simulink model "TRIGA_model"  (R2017b)
settings: Solver=ode15s  StartTime=0  StopTime=10000  RelTol=1e-2  EnableMultiTasking=on
values from neighbouring files (symbols this model uses):
  A_Frict = (H_Core*F_D)./(2*DEq*(AFlow^2)*Rho_In)    [ReactorModel.m]
  AFlow = 0.06352    [ReactorModel.m]
  Alpha_C = 4*10^-5    (= 4e-05)    [ReactorModel.m]
  Alpha_F = -8.5*10^-5    (= -8.5e-05)    [ReactorModel.m]
  Alpha_V = -2.5e-06    [ReactorModel.m]
  Beta = BetaTOT*Fraction    [ReactorModel.m]
  BetaTOT = 730*10^-5    (= 0.0073)    [ReactorModel.m]
  CCool = CCool*1000    [ReactorModel.m]
  DEq = 4*AFlow/PWet    (= 0.0237633472062)    [ReactorModel.m]
  ESigmaF = U_0*SigmaFiss    (= 0.056935026)    [ReactorModel.m]
  f = 1    [ReactorModel.m]
  GCore_0 = (H_Core*9.81*Rho_In*NuExp.*P0./(A_Frict.*CCool)).^(1/3)    [ReactorModel.m]
  H_Active = 0.381    [ReactorModel.m]
  H_Core = 0.7224    [ReactorModel.m]
  I_0 = (Y_I*SigmaFiss*U_0*Phi_0)/LambdaI    (= 1.16996991958e+14)    [ReactorModel.m]
  KCool = XSteam('tc_pT',Pressure,TCool_0)    [ReactorModel.m]
  Lambda = [3.01 1.14 0.301 0.111 0.0305 0.0124]    [ReactorModel.m]
  LambdaI = 2.87*10^-5    (= 2.87e-05)    [ReactorModel.m]
  LambdaPm = 3.63*10^-6    (= 3.63e-06)    [ReactorModel.m]
  LambdaXe = 2.09*10^-5    (= 2.09e-05)    [ReactorModel.m]
  Life = 60*10^-6    (= 6e-05)    [ReactorModel.m]
  M1 = 7    [ReactorModel.m]
  M3 = 7.6    [ReactorModel.m]
  M_Res = 800    [ReactorModel.m]
  MCool = 22.57    [ReactorModel.m]
  MPool = 18963    [ReactorModel.m]
  Mu = XSteam('my_pT', Pressure, TCool_0)    [ReactorModel.m]
  N_Fuel = 83    [ReactorModel.m]
  N_Mean = 2.43    [ReactorModel.m]
  NuExp = 245*10^-6    (= 0.000245)    [ReactorModel.m]
  P0 = 50000    [ReactorModel.m]
  Phi_0 = P0/(EFiss*ESigmaF*N_Fuel*V_Fuel*10^6)    (= 922945828545)    [ReactorModel.m]
  Pm_0 = (Y_Pm*SigmaFiss*U_0*Phi_0)/LambdaPm    (= 1.55038151024e+14)    [ReactorModel.m]
  Pr = (Mu.*CCool)./KCool    [ReactorModel.m]
  PWet = 2*pi*RCladO*91    (= 10.6920964372)    [ReactorModel.m]
  R_Rod = 0.00089    [ReactorModel.m]
  RCladO = 0.0187    [ReactorModel.m]
  Rho_0 = XSteam('rho_pT', Pressure, TCool_0)    [ReactorModel.m]
  RT_Clad = (log(RCladO/R_CladI))/(2*pi*K_Clad)    [ReactorModel.m]
  RT_Fuel = 1/(8*pi*K_Fuel)    (= 0.00226329555023)    [ReactorModel.m]
  RT_Gap = 1/(2*pi*R_GapO*H_Gap)    (= 0.00348193602083)    [ReactorModel.m]
  SigmaSm = 4.1*10^-20    (= 4.1e-20)    [ReactorModel.m]
  SigmaXe = 2.65*10^-18    (= 2.65e-18)    [ReactorModel.m]
  Sm_0 = (LambdaPm*Pm_0)/(SigmaSm*Phi_0)    (= 1.48725397185e+16)    [ReactorModel.m]
  Step = 1    [ReactorModel.m]
  T_Aq = 15    [ReactorModel.m]
  TCool_0 = TPool_0+(P0./(20*GCore_0.*CCool))    [ReactorModel.m]
  TFuel_0 = (f*P0./K)+TCool_0    [ReactorModel.m]
  TPool_0 = TPool_R+(P0./(MPool*CCool))    [ReactorModel.m]
  TPool_R = 20    [ReactorModel.m]
  W = 0.5    [ReactorModel.m]
  Xe_0 = (Y_Xe*SigmaFiss*U_0*Phi_0 + LambdaI*I_0)/(SigmaXe*Phi_0 + LambdaXe)    (= 1.49163932561e+14)    [ReactorModel.m]
  Y_I = 0.0639    [ReactorModel.m]
  Y_Pm = 0.01071    [ReactorModel.m]
  Y_Xe = 0.00237    [ReactorModel.m]
libraries: simulink x2
settings Model: Creator=dironco  LastModifiedBy=Introini Carolina
settings DataIOCC: LimitDataPoints=on  InspectSignalLogs=on
settings OptimizationCC: LifeSpan=inf
settings DebuggingCC: AllowSymbolicDim=off  SFUnexpectedBacktrackingDiag=warning  SFNoUnconditionalDefaultTransitionDiag=warning  SFExecutionAtInitializationDiag=none
settings ModelReferenceCC: PropagateSignalLabelsOutOfModel=off
settings CodeAppCC: StateflowObjectComments=on
settings GRTTargetCC: TargetLangStandard=C89/C90 (ANSI)
settings ConfigComp: CovMetricSettings=dw  CovHtmlReporting=on  CovSaveCumulativeToWorkspaceVar=on  CovSaveSingleToWorkspaceVar=on  CovExternalEMLEnable=off

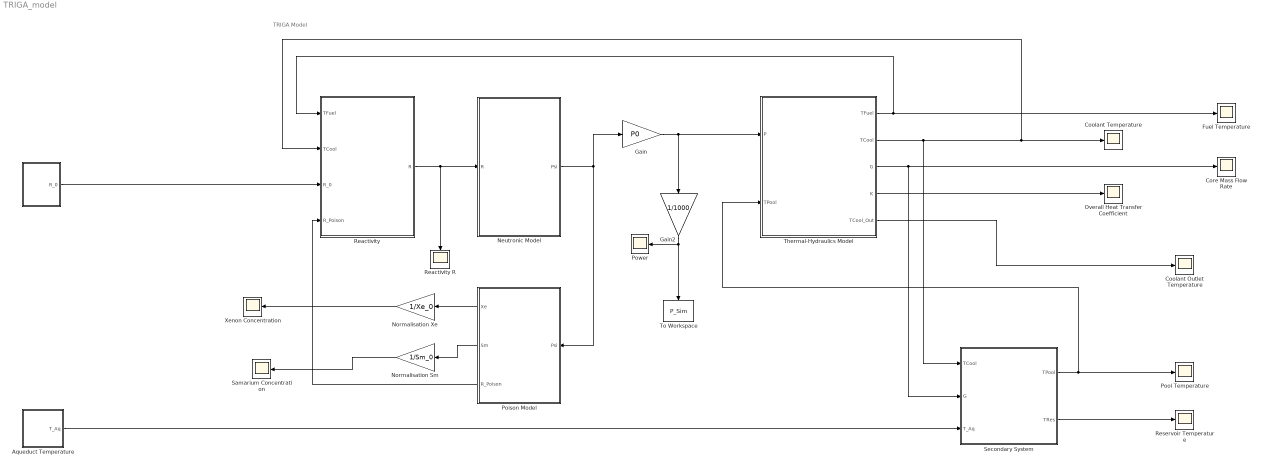
== system TRIGA_model ==
  note: TRIGA Model
  " " : Subsystem  Tag=Input Reactivity
  Aqueduct Temperature : Subsystem
  Coolant Outlet Temperature : Scope
  Coolant Temperature : Scope
  Core Mass Flow Rate : Scope
  Fuel Temperature : Scope
  Gain : Gain  Gain=P0
  Gain2 : Gain  Gain=1/1000
  Neutronic Model : Subsystem
  Normalisation Sm : Gain  Gain=1/Sm_0
  Normalisation Xe : Gain  Gain=1/Xe_0
  Overall Heat Transfer Coefficient : Scope
  Poison Model : Subsystem
  Pool Temperature : Scope
  Power : Scope
  Reactivity : Subsystem
  Reactivity R : Scope
  Reservoir Temperature : Scope
  Samarium Concentration : Scope
  Secondary System : Subsystem
  "Thermal-Hydraulics Model " : Subsystem
  To Workspace : ToWorkspace  VariableName=P_Sim  SaveFormat=Structure With Time  SampleTime=0.1
  Xenon Concentration : Scope
  wires:
  "Thermal-Hydraulics Model "/2(TCool) -> Secondary System/1(TCool), Reactivity/2(TCool), Coolant Temperature/1
  "Thermal-Hydraulics Model "/4(K) -> Overall Heat Transfer Coefficient/1
  Secondary System/1(TPool) -> "Thermal-Hydraulics Model "/2(TPool), Pool Temperature/1
  "Thermal-Hydraulics Model "/1(TFuel) -> Reactivity/1(TFuel), Fuel Temperature/1
  "Thermal-Hydraulics Model "/5(TCool_Out) -> Coolant Outlet Temperature/1
  "Thermal-Hydraulics Model "/3(G) -> Secondary System/2(G), Core Mass Flow Rate/1
  Gain2/1 -> To Workspace/1, Power/1
  Reactivity/1(R) -> Neutronic Model/1(R), Reactivity R/1
  Normalisation Xe/1 -> Xenon Concentration/1
  Normalisation Sm/1 -> Samarium Concentration/1
  Secondary System/2(TRes) -> Reservoir Temperature/1
  Poison Model/1(Xe) -> Normalisation Xe/1
  Poison Model/3(R_Poison) -> Reactivity/4(R_Poison)
  Aqueduct Temperature/1(T_Aq) -> Secondary System/3(T_Aq)
  " "/1(R_0) -> Reactivity/3(R_0)
  Poison Model/2(Sm) -> Normalisation Sm/1
  Gain/1 -> "Thermal-Hydraulics Model "/1(P), Gain2/1
  Neutronic Model/1("Psi ") -> Poison Model/1(Psi), Gain/1

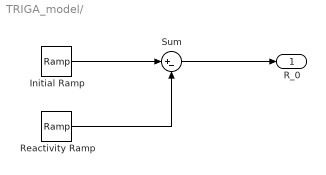
== system TRIGA_model/  ==
  Initial Ramp : simulink/Sources/Ramp  slope=R_Rod/Step  start=50  X0=0
  Reactivity Ramp : simulink/Sources/Ramp  slope=R_Rod/Step  start=Step+50  X0=0
  Sum : Sum  Inputs=|+-
  R_0 : Outport
  wires:
  Reactivity Ramp/1 -> Sum/2
  Initial Ramp/1 -> Sum/1
  Sum/1 -> R_0/1

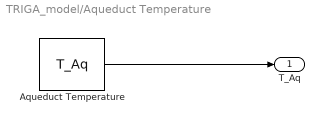
== system TRIGA_model/Aqueduct Temperature ==
  Aqueduct Temperature : Constant  Value=T_Aq
  T_Aq : Outport
  wires:
  Aqueduct Temperature/1 -> T_Aq/1

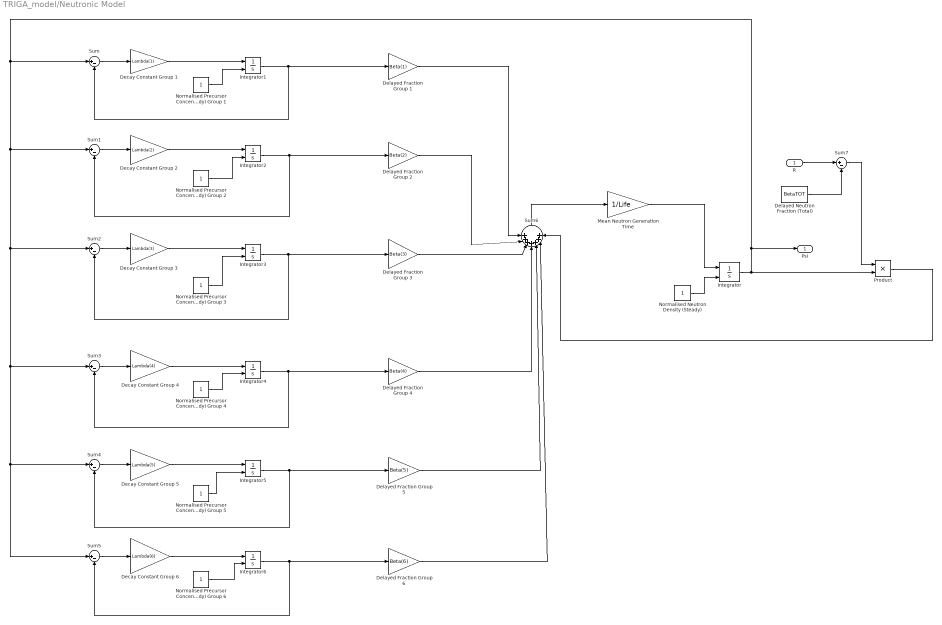
== system TRIGA_model/Neutronic Model ==
  R : Inport
  Decay Constant Group 1 : Gain  Gain=Lambda(1)
  Decay Constant Group 2 : Gain  Gain=Lambda(2)
  Decay Constant Group 3 : Gain  Gain=Lambda(3)
  Decay Constant Group 4 : Gain  Gain=Lambda(4)
  Decay Constant Group 5 : Gain  Gain=Lambda(5)
  Decay Constant Group 6 : Gain  Gain=Lambda(6)
  Delayed Fraction Group 1 : Gain  Gain=Beta(1)
  Delayed Fraction Group 2 : Gain  Gain=Beta(2)
  Delayed Fraction Group 3 : Gain  Gain=Beta(3)
  Delayed Fraction Group 4 : Gain  Gain=Beta(4)
  Delayed Fraction Group 5 : Gain  Gain=Beta(5)
  Delayed Fraction Group 6 : Gain  Gain=Beta(6)
  Delayed Neutron Fraction (Total) : Constant  Value=BetaTOT
  Integrator{,1..6} (7 alike) : Integrator  InitialConditionSource=external
  Mean Neutron Generation Time : Gain  Gain=1/Life
  Normalised Precursor Concentration (Steady) Group {1..6} (6 alike) : Constant
  Normalised Neutron Density (Steady) : Constant
  Product : Product
  Sum{,1..5,7} (7 alike) : Sum  Inputs=|+-
  Sum6 : Sum  Inputs=+++++++
  "Psi " : Outport
  wires:
  Sum1/1 -> Decay Constant Group 2/1
  Sum/1 -> Decay Constant Group 1/1
  Sum3/1 -> Decay Constant Group 4/1
  Sum5/1 -> Decay Constant Group 6/1
  Sum6/1 -> Mean Neutron Generation Time/1
  Integrator1/1 -> Sum/2, Delayed Fraction Group 1/1
  Integrator2/1 -> Sum1/2, Delayed Fraction Group 2/1
  Integrator3/1 -> Sum2/2, Delayed Fraction Group 3/1
  Sum4/1 -> Decay Constant Group 5/1
  Integrator4/1 -> Sum3/2, Delayed Fraction Group 4/1
  Sum2/1 -> Decay Constant Group 3/1
  Integrator5/1 -> Sum4/2, Delayed Fraction Group 5/1
  Delayed Fraction Group 5/1 -> Sum6/5
  Delayed Fraction Group 1/1 -> Sum6/1
  Mean Neutron Generation Time/1 -> Integrator/1
  Delayed Fraction Group 2/1 -> Sum6/2
  Delayed Fraction Group 4/1 -> Sum6/4
  Normalised Precursor Concentration (Steady) Group 5/1 -> Integrator5/2
  Integrator/1 -> Sum3/1, Sum5/1, Sum4/1, Sum2/1, Sum1/1, Sum/1, "Psi "/1, Product/2
  Normalised Precursor Concentration (Steady) Group 3/1 -> Integrator3/2
  Normalised Precursor Concentration (Steady) Group 2/1 -> Integrator2/2
  Normalised Precursor Concentration (Steady) Group 1/1 -> Integrator1/2
  Integrator6/1 -> Delayed Fraction Group 6/1, Sum5/2
  Delayed Fraction Group 6/1 -> Sum6/6
  Normalised Precursor Concentration (Steady) Group 6/1 -> Integrator6/2
  Normalised Precursor Concentration (Steady) Group 4/1 -> Integrator4/2
  Normalised Neutron Density (Steady)/1 -> Integrator/2
  Product/1 -> Sum6/7
  Delayed Fraction Group 3/1 -> Sum6/3
  R/1 -> Sum7/1
  Decay Constant Group 1/1 -> Integrator1/1
  Decay Constant Group 2/1 -> Integrator2/1
  Decay Constant Group 3/1 -> Integrator3/1
  Decay Constant Group 4/1 -> Integrator4/1
  Decay Constant Group 5/1 -> Integrator5/1
  Decay Constant Group 6/1 -> Integrator6/1
  Delayed Neutron Fraction (Total)/1 -> Sum7/2
  Sum7/1 -> Product/1

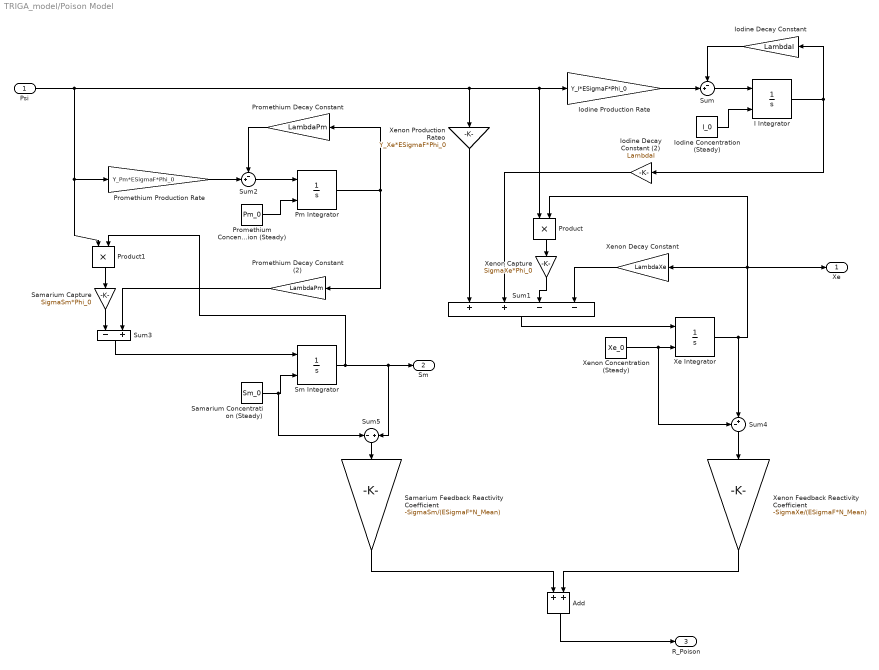
== system TRIGA_model/Poison Model ==
  Psi : Inport
  Add : Sum
  I Integrator : Integrator  InitialConditionSource=external
  Iodine Concentration (Steady) : Constant  Value=I_0
  Iodine Decay Constant : Gain  Gain=LambdaI
  Iodine Decay Constant (2) : Gain  Gain=LambdaI
  Iodine Production Rate : Gain  Gain=Y_I*ESigmaF*Phi_0
  Pm Integrator : Integrator  InitialConditionSource=external
  Product : Product
  Product1 : Product
  Promethium Concentration (Steady) : Constant  Value=Pm_0
  Promethium Decay Constant : Gain  Gain=LambdaPm
  Promethium Decay Constant (2) : Gain  Gain=LambdaPm
  "Promethium Production Rate " : Gain  Gain=Y_Pm*ESigmaF*Phi_0
  Samarium Capture : Gain  Gain=SigmaSm*Phi_0
  Samarium Concentration (Steady) : Constant  Value=Sm_0
  Samarium Feedback Reactivity Coefficient : Gain  Gain=-SigmaSm/(ESigmaF*N_Mean)
  Sm Integrator : Integrator  InitialConditionSource=external
  Sum : Sum  Inputs=-+|
  Sum1 : Sum  Inputs=++--
  Sum2 : Sum  Inputs=-+|
  Sum3 : Sum  Inputs=-+
  Sum4 : Sum  Inputs=-+|
  Sum5 : Sum  Inputs=-+
  Xe Integrator : Integrator  InitialConditionSource=external
  Xenon Capture : Gain  Gain=SigmaXe*Phi_0
  Xenon Feedback Reactivity Coefficient : Gain  Gain=-SigmaXe/(ESigmaF*N_Mean)
  Xenon Production Rateo : Gain  Gain=Y_Xe*ESigmaF*Phi_0
  Xenon Concentration (Steady) : Constant  Value=Xe_0
  Xenon Decay Constant : Gain  Gain=LambdaXe
  Xe : Outport
  Sm : Outport  Port=2
  R_Poison : Outport  Port=3
  wires:
  I Integrator/1 -> Iodine Decay Constant/1, Iodine Decay Constant (2)/1
  Iodine Decay Constant/1 -> Sum/1
  Iodine Concentration (Steady)/1 -> I Integrator/2
  Sum/1 -> I Integrator/1
  Iodine Production Rate/1 -> Sum/2
  Xe Integrator/1 -> Xe/1, Product/2, Xenon Decay Constant/1, Sum4/2
  Xenon Decay Constant/1 -> Sum1/4
  Sum1/1 -> Xe Integrator/1
  Iodine Decay Constant (2)/1 -> Sum1/2
  Xenon Production Rateo/1 -> Sum1/1
  Product/1 -> Xenon Capture/1
  Xenon Capture/1 -> Sum1/3
  Promethium Concentration (Steady)/1 -> Pm Integrator/2
  Psi/1 -> Iodine Production Rate/1, Product/1, Xenon Production Rateo/1, "Promethium Production Rate "/1, Product1/1
  Sum2/1 -> Pm Integrator/1
  Pm Integrator/1 -> Promethium Decay Constant (2)/1, Promethium Decay Constant/1
  Promethium Decay Constant/1 -> Sum2/1
  "Promethium Production Rate "/1 -> Sum2/2
  Sum3/1 -> Sm Integrator/1
  Promethium Decay Constant (2)/1 -> Sum3/2
  Product1/1 -> Samarium Capture/1
  Samarium Capture/1 -> Sum3/1
  Sm Integrator/1 -> Sum5/2, Sm/1, Product1/2
  Samarium Concentration (Steady)/1 -> Sum5/1, Sm Integrator/2
  Sum4/1 -> Xenon Feedback Reactivity Coefficient/1
  Xenon Concentration (Steady)/1 -> Sum4/1, Xe Integrator/2
  Sum5/1 -> Samarium Feedback Reactivity Coefficient/1
  Xenon Feedback Reactivity Coefficient/1 -> Add/2
  Samarium Feedback Reactivity Coefficient/1 -> Add/1
  Add/1 -> R_Poison/1

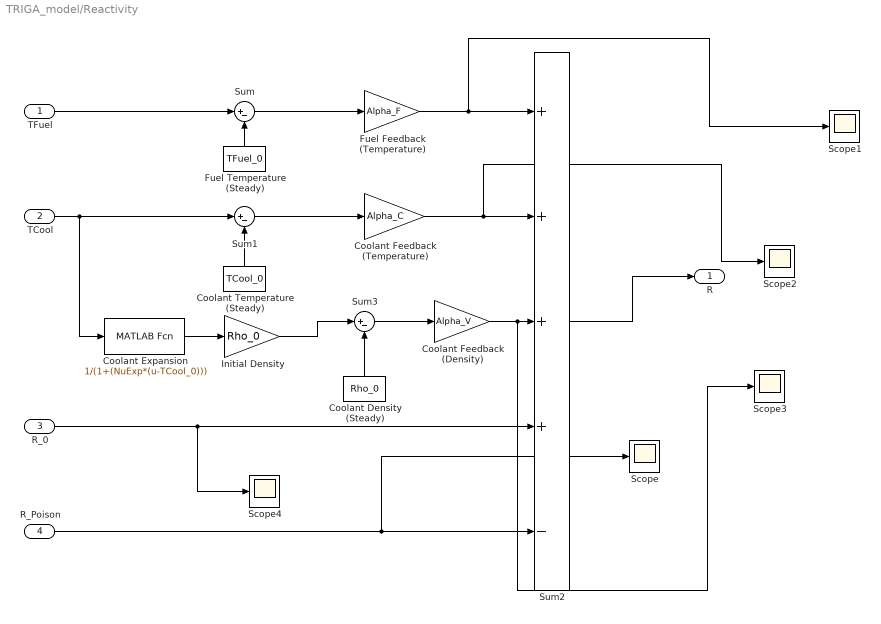
== system TRIGA_model/Reactivity ==
  TFuel : Inport
  TCool : Inport  Port=2
  R_0 : Inport  Port=3
  R_Poison : Inport  Port=4
  Coolant Density (Steady) : Constant  Value=Rho_0
  Coolant Expansion : MATLABFcn  MATLABFcn=1/(1+(NuExp*(u-TCool_0)))
  Coolant Feedback (Density) : Gain  Gain=Alpha_V
  Coolant Feedback (Temperature) : Gain  Gain=Alpha_C
  Coolant Temperature (Steady) : Constant  Value=TCool_0
  Fuel Feedback (Temperature) : Gain  Gain=Alpha_F
  Fuel Temperature (Steady) : Constant  Value=TFuel_0
  Initial Density : Gain  Gain=Rho_0
  Scope{,1..4} (5 alike) : Scope
  Sum : Sum  Inputs=|+-
  Sum1 : Sum  Inputs=|+-
  Sum2 : Sum  Inputs=++++-
  Sum3 : Sum  Inputs=|+-
  R : Outport
  wires:
  Coolant Temperature (Steady)/1 -> Sum1/2
  Sum2/1 -> R/1
  Sum1/1 -> Coolant Feedback (Temperature)/1
  TFuel/1 -> Sum/1
  Sum/1 -> Fuel Feedback (Temperature)/1
  R_0/1 -> Scope4/1, Sum2/4
  Coolant Feedback (Temperature)/1 -> Scope2/1, Sum2/2
  TCool/1 -> Coolant Expansion/1, Sum1/1
  Fuel Temperature (Steady)/1 -> Sum/2
  Fuel Feedback (Temperature)/1 -> Scope1/1, Sum2/1
  R_Poison/1 -> Scope/1, Sum2/5
  Coolant Feedback (Density)/1 -> Scope3/1, Sum2/3
  Coolant Expansion/1 -> Initial Density/1
  Initial Density/1 -> Sum3/1
  Sum3/1 -> Coolant Feedback (Density)/1
  Coolant Density (Steady)/1 -> Sum3/2

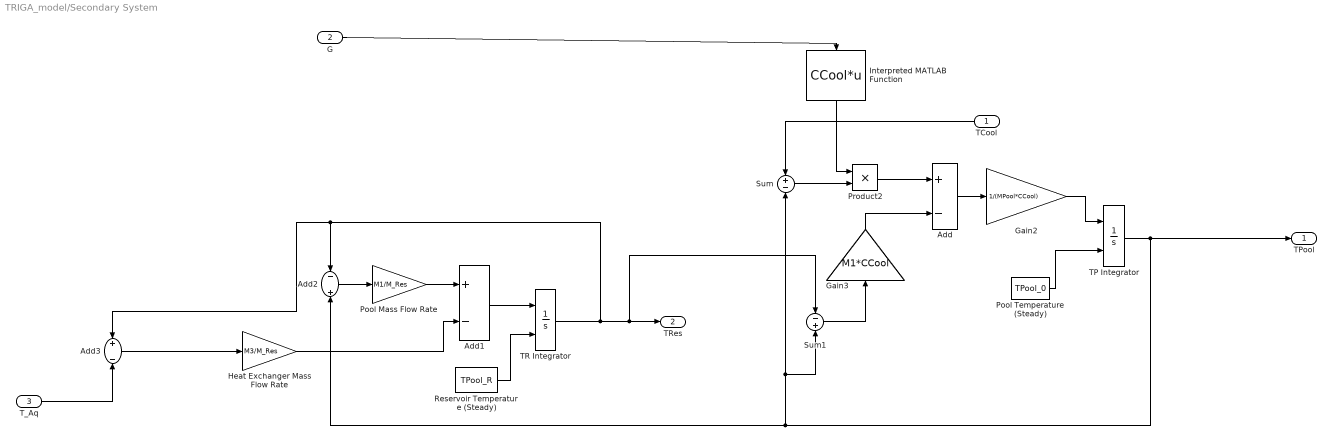
== system TRIGA_model/Secondary System ==
  TCool : Inport
  G : Inport  Port=2
  T_Aq : Inport  Port=3
  Add : Sum  Inputs=+-
  Add1 : Sum  Inputs=+-
  Add2 : Sum  Inputs=-+
  Add3 : Sum  Inputs=+-
  Gain2 : Gain  Gain=1/(MPool*CCool)
  Gain3 : Gain  Gain=M1*CCool
  "Heat Exchanger Mass Flow Rate " : Gain  Gain=M3/M_Res
  Interpreted MATLAB Function : MATLABFcn  MATLABFcn=CCool*u
  Pool Mass Flow Rate : Gain  Gain=M1/M_Res
  Pool Temperature (Steady) : Constant  Value=TPool_0
  Product2 : Product
  Reservoir Temperature (Steady) : Constant  Value=TPool_R
  Sum : Sum  Inputs=+-
  Sum1 : Sum  Inputs=-+
  TP Integrator : Integrator  InitialConditionSource=external
  TR Integrator : Integrator  InitialConditionSource=external
  TPool : Outport
  TRes : Outport  Port=2
  wires:
  Add1/1 -> TR Integrator/1
  Reservoir Temperature (Steady)/1 -> TR Integrator/2
  "Heat Exchanger Mass Flow Rate "/1 -> Add1/2
  Pool Temperature (Steady)/1 -> TP Integrator/2
  Gain2/1 -> TP Integrator/1
  Add3/1 -> "Heat Exchanger Mass Flow Rate "/1
  Interpreted MATLAB Function/1 -> Product2/1
  Add2/1 -> Pool Mass Flow Rate/1
  Pool Mass Flow Rate/1 -> Add1/1
  T_Aq/1 -> Add3/2
  G/1 -> Interpreted MATLAB Function/1
  Add/1 -> Gain2/1
  TP Integrator/1 -> TPool/1, Add2/2, Sum1/2, Sum/2
  TCool/1 -> Sum/1
  Sum/1 -> Product2/2
  Product2/1 -> Add/1
  Gain3/1 -> Add/2
  Sum1/1 -> Gain3/1
  TR Integrator/1 -> Sum1/1, TRes/1, Add3/1, Add2/1

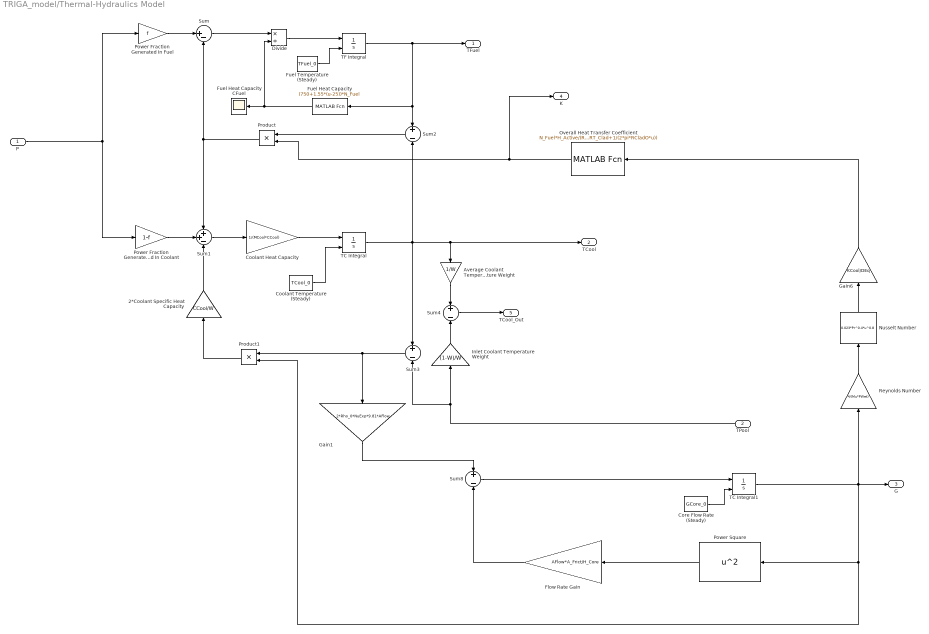
== system TRIGA_model/Thermal-Hydraulics Model  ==
  P : Inport
  TPool : Inport  Port=2
  2*Coolant Specific Heat Capacity : Gain  Gain=CCool/W
  Average Coolant Temperature Weight : Gain  Gain=1/W
  Coolant Heat Capacity : Gain  Gain=1/(MCool*CCool)
  Coolant Temperature (Steady) : Constant  Value=TCool_0
  Core Flow Rate (Steady) : Constant  Value=GCore_0
  Divide : Product  Inputs=*/
  Flow Rate Gain : Gain  Gain=AFlow*A_Frict/H_Core
  Fuel Heat Capacity CFuel : Scope
  Fuel Heat Capacity : MATLABFcn  MATLABFcn=(750+1.55*(u-25))*N_Fuel
  Fuel Temperature (Steady) : Constant  Value=TFuel_0
  Gain1 : Gain  Gain=2*Rho_0*NuExp*9.81*AFlow
  Gain6 : Gain  Gain=KCool/DEq
  Inlet Coolant Temperature Weight : Gain  Gain=(1-W)/W
  Nusselt Number : MATLABFcn  MATLABFcn=0.023*Pr^0.4*u^0.8
  Overall Heat Transfer Coefficient : MATLABFcn  MATLABFcn=N_Fuel*H_Active/(RT_Fuel+RT_Gap+RT_Clad+1/(2*pi*RCladO*u))
  Power Fraction Generated In Coolant : Gain  Gain=1-f
  Power Fraction Generated In Fuel : Gain  Gain=f
  Power Square : MATLABFcn  MATLABFcn=u^2
  Product : Product
  Product1 : Product
  Reynolds Number : Gain  Gain=4/(Mu*PWet)
  Sum : Sum  Inputs=|+-
  Sum1 : Sum  Inputs=++-
  Sum{2..4,8} (4 alike) : Sum  Inputs=+-
  TC Integral : Integrator  InitialConditionSource=external
  TC Integral1 : Integrator  InitialConditionSource=external
  TF Integral : Integrator  InitialConditionSource=external
  TFuel : Outport
  TCool : Outport  Port=2
  G : Outport  Port=3
  K : Outport  Port=4
  TCool_Out : Outport  Port=5
  wires:
  TC Integral/1 -> Sum3/1, TCool/1, Average Coolant Temperature Weight/1, Sum2/2
  Product/1 -> Sum1/1, Sum/2
  Sum2/1 -> Product/1
  TF Integral/1 -> TFuel/1, Sum2/1, Fuel Heat Capacity/1
  Power Fraction Generated In Fuel/1 -> Sum/1
  Power Fraction Generated In Coolant/1 -> Sum1/2
  Sum1/1 -> Coolant Heat Capacity/1
  P/1 -> Power Fraction Generated In Coolant/1, Power Fraction Generated In Fuel/1
  Fuel Temperature (Steady)/1 -> TF Integral/2
  Coolant Temperature (Steady)/1 -> TC Integral/2
  Coolant Heat Capacity/1 -> TC Integral/1
  2*Coolant Specific Heat Capacity/1 -> Sum1/3
  Product1/1 -> 2*Coolant Specific Heat Capacity/1
  Overall Heat Transfer Coefficient/1 -> Product/2, K/1
  Divide/1 -> TF Integral/1
  Sum/1 -> Divide/1
  Fuel Heat Capacity/1 -> Divide/2, Fuel Heat Capacity CFuel/1
  Nusselt Number/1 -> Gain6/1
  Reynolds Number/1 -> Nusselt Number/1
  Gain6/1 -> Overall Heat Transfer Coefficient/1
  Average Coolant Temperature Weight/1 -> Sum4/1
  Inlet Coolant Temperature Weight/1 -> Sum4/2
  Sum4/1 -> TCool_Out/1
  Sum3/1 -> Product1/1, Gain1/1
  TC Integral1/1 -> Reynolds Number/1, Product1/2, Power Square/1, G/1
  Core Flow Rate (Steady)/1 -> TC Integral1/2
  Gain1/1 -> Sum8/1
  Sum8/1 -> TC Integral1/1
  Flow Rate Gain/1 -> Sum8/2
  Power Square/1 -> Flow Rate Gain/1
  TPool/1 -> Inlet Coolant Temperature Weight/1, Sum3/2
